simulink model "PendulumCartOL"  (Simulink 8.4)
settings: Solver=ode45  StartTime=0.0  StopTime=10  MinStep=1E-2  RelTol=1e-4
values from neighbouring files (symbols this model uses):
  A = [zeros(2) eye(2); -inv(M)*kappa -inv(M)*beta]    [Lab3_Solution.m]    (also in lab4.m = [0 0 1 0; 0 0 0 1; 0 (mp^2 * l^2 *g)/mu (-c*Jt)/mu (-Y*Jt*l*; lab4_pid_controller.m; lab4_state_feedback_no_estimator.m; lab4_state_feedback_with_estimator.m)
  B = [0; 0; inv(M)*S]    [Lab3_Solution.m]    (also in lab4.m = [0; 0; Jt/mu; (l*mp)/mu]; lab4_pid_controller.m; lab4_state_feedback_no_estimator.m; lab4_state_feedback_with_estimator.m)
  C = [1 0 0 0; 0 1 0 0]    [Lab3_Solution.m]    (also in PendulumTutorial.m = zpk(z,p,k); lab4.m; lab4_pid_controller.m; lab4_state_feedback_no_estimator.m = eye(4))
  D = [0; 0]    [Lab3_Solution.m]    (also in lab4.m; lab4_pid_controller.m; lab4_state_feedback_no_estimator.m = [0; 0; 0; 0]; lab4_state_feedback_with_estimator.m)
libraries: simulink_extras x1
settings Model: Creator=johnchipoco  LastModifiedBy=vincentchow
settings DataIOCC: SignalLoggingSaveFormat=Dataset
settings OptimizationCC: ExpressionDepthLimit=128
settings DebuggingCC: UnderspecifiedInitializationDetection=Simplified  MergeDetectMultiDrivingBlocksExec=error  FcnCallInpInsideContextMsg=EnableAllAsError  StateNameClashWarn=none
settings GRTTargetCC: CombineOutputUpdateFcns=on  GRTInterface=off

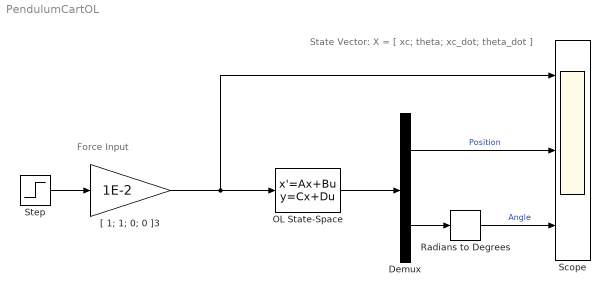
== system PendulumCartOL ==
  note: Force Input
  note: State Vector: X = [ xc; theta; xc_dot; theta_dot ]
  Demux : Demux  Outputs=2
  OL State-Space : StateSpace  A=A  B=B  C=C  D=D  X0=[0; 0; 0; 0 ]
  Radians to Degrees : simulink_extras/Transformations/Radians to Degrees
  Scope : Scope  NumInputPorts=3
      settings: TickLabels=on  TimeRange=10  YMin=0~-0.012~-0.2  YMax=0.1~0~1.4  SaveName=FSR_data
  Step : Step  Time=0.5  SampleTime=0
  "[ 1; 1; 0; 0 ]3" : Gain  Gain=1E-2  SaturateOnIntegerOverflow=on  OutDataTypeStr=Inherit: Same as input  ParamDataTypeStr=Inherit: Same as input
  wires:
  Demux/2 -> Radians to Degrees/1
  "[ 1; 1; 0; 0 ]3"/1 -> OL State-Space/1, Scope/1
  Step/1 -> "[ 1; 1; 0; 0 ]3"/1
  OL State-Space/1 -> Demux/1
  Demux/1 -> Scope/2  "Position"
  Radians to Degrees/1 -> Scope/3  "Angle"
